simulink model "Third"  (R2021b)
settings: Solver=VariableStepAuto  StartTime=0.0  StopTime=150  RelTol=1e-3
values from neighbouring files (symbols this model uses):
  alpha0 = trim_state_lo(8)    [Glideslope.m]
  coeff_x = x0/sqrt(x0^2+y0^2)    [Glideslope.m]
  coeff_y = y0/sqrt(x0^2+y0^2)    [Glideslope.m]
  h_flare = 19.1817    [Glideslope.m]
  max_dev_elevator = 25 - trim_control_lo(1)    [Glideslope.m]
  max_dev_thrust = 19000 - trim_thrust_lo    [Glideslope.m]
  min_dev_elevator = -25 - trim_control_lo(1)    [Glideslope.m]
  min_dev_thrust = 1000 - trim_thrust_lo    [Glideslope.m]
  tau = 1.2217    [Glideslope.m]
  theta0 = trim_state_lo(5)    [Glideslope.m]
  x0 = 3000 + 2000/(3*pi/180)    (= 41197.1863421)    [Glideslope.m]
undefined symbols (not defined in the file or in its folder): magnitude
libraries: slpidlib x2, cstblocks x1
settings Model: Creator=misha  LastModifiedBy=ddefu

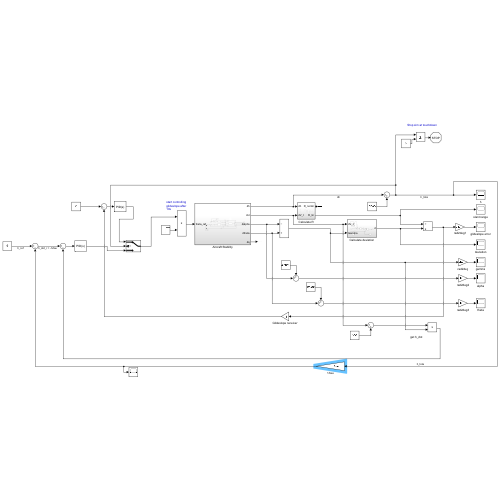
[thumbnail: Simulink's stored preview of the top-level diagram]
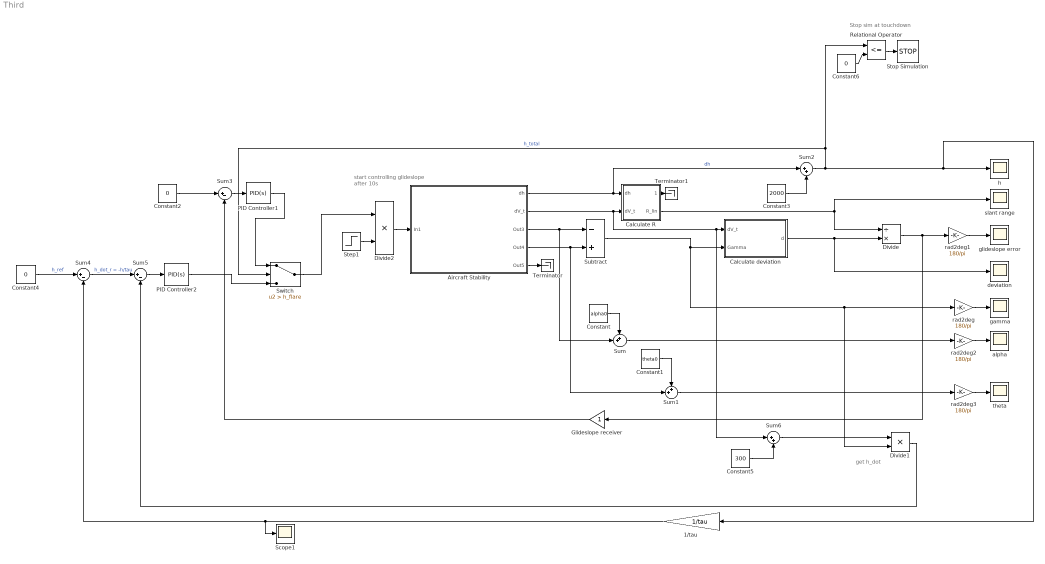
== system Third ==
  note: Stop sim at touchdown
  note: get h_dot
  note: start controlling glideslope after 10s
  1/tau : Gain  Gain=1/tau
  Aircraft Stability : Subsystem
  Calculate R : Subsystem
  Calculate deviation : Subsystem
  Constant : Constant  Value=alpha0
  Constant1 : Constant  Value=theta0
  Constant2 : Constant  Value=0
  Constant3 : Constant  Value=2000
  Constant4 : Constant  Value=0
  Constant5 : Constant  Value=300
  Constant6 : Constant  Value=0
  Divide : Product  Inputs=/*
  Divide1 : Product  Inputs=**
  Divide2 : Product  Inputs=**
  Glideslope receiver : Gain
  PID Controller1 : slpidlib/PID Controller  Controller=PID  Form=Parallel  TimeDomain=Continuous-time  UseExternalTs=off  SampleTime=-1  IntegratorMethod=Forward Euler  FilterMethod=Forward Euler  ControllerParametersSource=internal  P=2000  I=200  D=0  UseFilter=on  N=100  TunerSelectOption=Transfer Function Based (PID Tuner App)  InitialConditionSource=internal  InitialConditionForIntegrator=0  InitialConditionForFilter=0  DifferentiatorICPrevScaledInput=0  ExternalReset=none  TrackingMode=off  Kt=1  LimitOutput=off  SatLimitsSource=internal  UpperSaturationLimit=inf  LowerSaturationLimit=-inf  LinearizeAsGain=on  AntiWindupMode=none  Kb=1  POutMin=[]  POutMax=[]  IOutMin=[]  IOutMax=[]  DOutMin=[]  DOutMax=[]  NOutMin=[]  NOutMax=[]  SumOutMin=[]  SumOutMax=[]  SaturationOutMin=[]  SaturationOutMax=[]  PParamMin=[]  PParamMax=[]  IParamMin=[]  IParamMax=[]  DParamMin=[]  DParamMax=[]  NParamMin=[]  NParamMax=[]  KbParamMin=[]  KbParamMax=[]  KtParamMin=[]  KtParamMax=[]  KbOutMin=[]  KbOutMax=[]  KtOutMin=[]  KtOutMax=[]  IntegratorOutMin=[]  IntegratorOutMax=[]  FilterOutMin=[]  FilterOutMax=[]  SumI1OutMin=[]  SumI1OutMax=[]  SumI2OutMin=[]  SumI2OutMax=[]  SumI3OutMin=[]  SumI3OutMax=[]  SumI4OutMin=[]  SumI4OutMax=[]  SumDOutMin=[]  SumDOutMax=[]  DifferentiatorOutMin=[]  DifferentiatorOutMax=[]  FilterDiffOutCoefMin=[]  FilterDiffOutCoefMax=[]  ReciprocalOutMin=[]  ReciprocalOutMax=[]  SumDenOutMin=[]  SumDenOutMax=[]  SumNumOutMin=[]  SumNumOutMax=[]  DivideOutMin=[]  DivideOutMax=[]  UdiffTsProdOutMin=[]  UdiffTsProdOutMax=[]  NTsProdOutMin=[]  NTsProdOutMax=[]  UintegralTsProdOutMin=[]  UintegralTsProdOutMax=[]  UngainTsProdOutMin=[]  UngainTsProdOutMax=[]  IntegratorContinuousStateAttributes=''  IntegratorStateMustResolveToSignalObject=off  IntegratorRTWStateStorageClass=Auto  FilterContinuousStateAttributes=''  FilterStateMustResolveToSignalObject=off  FilterRTWStateStorageClass=Auto  ParallelPVariant=InternalParameters  IdealPVariant=Disabled  IVariant=InternalParameters  DVariant=InternalParameters  IntegratorVariant=Continuous  SatVariant=Disabled  AWVariant=Passthrough  PCopyVariant=Disabled  TRVariant=Disabled  FdbkBlocksVariant=Forward  IdealPFdbkVariant=Disabled  SatFdbkVariant=Disabled  DerivativeFilterVariant=ContFilter  NVariant=InternalParameters  NCopyVariant=Disabled  FilterICVariant=InternalICsFilter  IntegratorICVariant=InternalICs  ExternalResetVariant=Disabled  TRSumVariant=Passthrough  SumFdbkVariant=Disabled  SumVariant=Sum_PID  TsampFilterVariant=InternalTs  TsampNgainVariant=Passthrough  TsampIntegralVariant=Passthrough  ExternalSaturationOutDataTypeStr=Inherit: Same as second input
  PID Controller2 : slpidlib/PID Controller  Controller=PID  Form=Parallel  TimeDomain=Continuous-time  UseExternalTs=off  SampleTime=-1  IntegratorMethod=Forward Euler  FilterMethod=Forward Euler  ControllerParametersSource=internal  P=2000  I=200  D=0  UseFilter=on  N=100  TunerSelectOption=Transfer Function Based (PID Tuner App)  InitialConditionSource=internal  InitialConditionForIntegrator=0  InitialConditionForFilter=0  DifferentiatorICPrevScaledInput=0  ExternalReset=none  TrackingMode=off  Kt=1  LimitOutput=off  SatLimitsSource=internal  UpperSaturationLimit=inf  LowerSaturationLimit=-inf  LinearizeAsGain=on  AntiWindupMode=none  Kb=1  POutMin=[]  POutMax=[]  IOutMin=[]  IOutMax=[]  DOutMin=[]  DOutMax=[]  NOutMin=[]  NOutMax=[]  SumOutMin=[]  SumOutMax=[]  SaturationOutMin=[]  SaturationOutMax=[]  PParamMin=[]  PParamMax=[]  IParamMin=[]  IParamMax=[]  DParamMin=[]  DParamMax=[]  NParamMin=[]  NParamMax=[]  KbParamMin=[]  KbParamMax=[]  KtParamMin=[]  KtParamMax=[]  KbOutMin=[]  KbOutMax=[]  KtOutMin=[]  KtOutMax=[]  IntegratorOutMin=[]  IntegratorOutMax=[]  FilterOutMin=[]  FilterOutMax=[]  SumI1OutMin=[]  SumI1OutMax=[]  SumI2OutMin=[]  SumI2OutMax=[]  SumI3OutMin=[]  SumI3OutMax=[]  SumI4OutMin=[]  SumI4OutMax=[]  SumDOutMin=[]  SumDOutMax=[]  DifferentiatorOutMin=[]  DifferentiatorOutMax=[]  FilterDiffOutCoefMin=[]  FilterDiffOutCoefMax=[]  ReciprocalOutMin=[]  ReciprocalOutMax=[]  SumDenOutMin=[]  SumDenOutMax=[]  SumNumOutMin=[]  SumNumOutMax=[]  DivideOutMin=[]  DivideOutMax=[]  UdiffTsProdOutMin=[]  UdiffTsProdOutMax=[]  NTsProdOutMin=[]  NTsProdOutMax=[]  UintegralTsProdOutMin=[]  UintegralTsProdOutMax=[]  UngainTsProdOutMin=[]  UngainTsProdOutMax=[]  IntegratorContinuousStateAttributes=''  IntegratorStateMustResolveToSignalObject=off  IntegratorRTWStateStorageClass=Auto  FilterContinuousStateAttributes=''  FilterStateMustResolveToSignalObject=off  FilterRTWStateStorageClass=Auto  ParallelPVariant=InternalParameters  IdealPVariant=Disabled  IVariant=InternalParameters  DVariant=InternalParameters  IntegratorVariant=Continuous  SatVariant=Disabled  AWVariant=Passthrough  PCopyVariant=Disabled  TRVariant=Disabled  FdbkBlocksVariant=Forward  IdealPFdbkVariant=Disabled  SatFdbkVariant=Disabled  DerivativeFilterVariant=ContFilter  NVariant=InternalParameters  NCopyVariant=Disabled  FilterICVariant=InternalICsFilter  IntegratorICVariant=InternalICs  ExternalResetVariant=Disabled  TRSumVariant=Passthrough  SumFdbkVariant=Disabled  SumVariant=Sum_PID  TsampFilterVariant=InternalTs  TsampNgainVariant=Passthrough  TsampIntegralVariant=Passthrough  ExternalSaturationOutDataTypeStr=Inherit: Same as second input
  Relational Operator : RelationalOperator  Operator=<=  OutDataTypeStr=boolean  RndMeth=Simplest
  Scope1 : Scope
  Step1 : Step  Time=10  SampleTime=0
  Stop Simulation : Stop
  Subtract : Sum  Inputs=-+
  Sum : Sum  Inputs=++|
  Sum1 : Sum  Inputs=++|
  Sum2 : Sum  Inputs=|++
  Sum3 : Sum  Inputs=|+-
  Sum4 : Sum  Inputs=|+-
  Sum5 : Sum  Inputs=|+-
  Sum6 : Sum  Inputs=|++
  Switch : Switch  Criteria=u2 > Threshold  Threshold=h_flare
  Terminator : Terminator
  Terminator1 : Terminator
  alpha : Scope
  deviation : Scope
  gamma : Scope
  glideslope error : Scope
  h : Scope
  rad2deg{,1..3} (4 alike) : Gain  Gain=180/pi
  slant range : Scope
  theta : Scope
  wires:
  Aircraft Stability/1(dh) -> Sum2/1, Calculate R/1(dh)  "dh"
  Aircraft Stability/2(dV_t) -> Sum6/1, Calculate deviation/1(dV_t), Calculate R/2(dV_t)
  Aircraft Stability/4(Out4) -> Sum1/2, Subtract/2
  Aircraft Stability/5(Out5) -> Terminator/1
  Divide/1 -> Glideslope receiver/1, rad2deg1/1
  Glideslope receiver/1 -> Sum3/2
  Constant2/1 -> Sum3/1
  Subtract/1 -> Calculate deviation/2(Gamma), rad2deg/1, Divide1/2
  Sum3/1 -> PID Controller1/1
  Aircraft Stability/3(Out3) -> Subtract/1, Sum/2
  PID Controller1/1 -> Switch/1
  Step1/1 -> Divide2/2
  Divide2/1 -> Aircraft Stability/1(In1)
  rad2deg/1 -> gamma/1
  rad2deg1/1 -> glideslope error/1
  Calculate deviation/1(d) -> Divide/2, deviation/1
  Calculate R/1(R_nonlin) -> Terminator1/1
  Calculate R/2(R_lin) -> Divide/1, slant range/1
  Constant/1 -> Sum/1
  Constant1/1 -> Sum1/1
  rad2deg2/1 -> alpha/1
  rad2deg3/1 -> theta/1
  Sum/1 -> rad2deg2/1
  Sum1/1 -> rad2deg3/1
  Constant3/1 -> Sum2/2
  Sum2/1 -> Relational Operator/1, Switch/2, 1/tau/1, h/1  "h_total"
  Constant4/1 -> Sum4/1  "h_ref"
  1/tau/1 -> Scope1/1, Sum4/2
  Sum4/1 -> Sum5/1  "h_dot_r = -h/tau"
  Constant5/1 -> Sum6/2
  Sum6/1 -> Divide1/1
  Divide1/1 -> Sum5/2
  Sum5/1 -> PID Controller2/1
  Relational Operator/1 -> Stop Simulation/1
  Constant6/1 -> Relational Operator/2
  Switch/1 -> Divide2/1
  PID Controller2/1 -> Switch/3

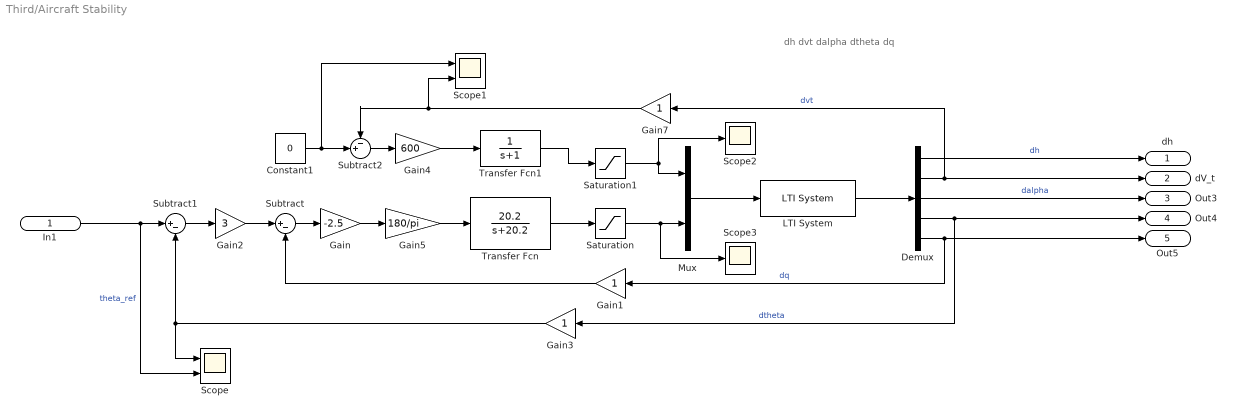
== system Third/Aircraft Stability ==
  note: dh
      | dvt
      | dalpha
      | dtheta
      | dq
  In1 : Inport
  Constant1 : Constant  Value=0
  Demux : Demux  Outputs=5
  Gain : Gain  Gain=-2.5
  Gain1 : Gain
  Gain2 : Gain  Gain=3
  Gain3 : Gain
  Gain4 : Gain  Gain=600
  Gain5 : Gain  Gain=180/pi
  Gain7 : Gain
  LTI System : cstblocks/LTI System  sys=sys_reduced  IC=[]
  Mux : Mux  Inputs=2
  Saturation : Saturate  UpperLimit=max_dev_elevator  LowerLimit=min_dev_elevator
  Saturation1 : Saturate  UpperLimit=max_dev_thrust  LowerLimit=min_dev_thrust
  Scope : Scope  NumInputPorts=2
  Scope1 : Scope  NumInputPorts=2
  Scope2 : Scope
  Scope3 : Scope
  Subtract : Sum  Inputs=|+-
  Subtract1 : Sum  Inputs=|+-
  Subtract2 : Sum  Inputs=-+|
  Transfer Fcn : TransferFcn  Numerator=[20.2]  Denominator=[1 20.2]
  Transfer Fcn1 : TransferFcn  Denominator=[1 1]
  dh : Outport
  dV_t : Outport  Port=2
  Out3 : Outport  Port=3
  Out4 : Outport  Port=4
  Out5 : Outport  Port=5
  wires:
  Gain5/1 -> Transfer Fcn/1
  In1/1 -> Subtract1/1, Scope/2  "theta_ref"
  Demux/4 -> Out4/1, Gain3/1  "dtheta"
  Gain2/1 -> Subtract/1
  Gain/1 -> Gain5/1
  Mux/1 -> LTI System/1
  Gain1/1 -> Subtract/2
  Gain3/1 -> Subtract1/2, Scope/1
  Saturation/1 -> Mux/2, Scope3/1
  Transfer Fcn1/1 -> Saturation1/1
  LTI System/1 -> Demux/1
  Saturation1/1 -> Scope2/1, Mux/1
  Demux/3 -> Out3/1  "dalpha"
  Demux/2 -> dV_t/1, Gain7/1  "dvt"
  Demux/5 -> Gain1/1, Out5/1  "dq"
  Subtract/1 -> Gain/1
  Constant1/1 -> Scope1/1, Subtract2/2
  Gain7/1 -> Scope1/2, Subtract2/1
  Demux/1 -> dh/1  "dh"
  Subtract1/1 -> Gain2/1
  Transfer Fcn/1 -> Saturation/1
  Subtract2/1 -> Gain4/1
  Gain4/1 -> Transfer Fcn1/1

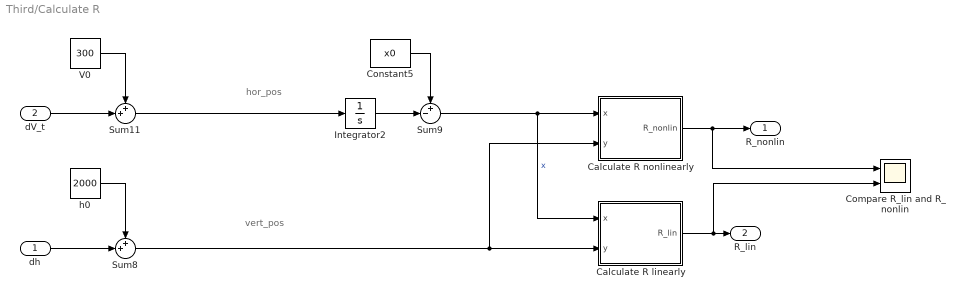
== system Third/Calculate R ==
  note: vert_pos
  note: hor_pos
  dh : Inport
  dV_t : Inport  Port=2
  Calculate R linearly : Subsystem
  Calculate R nonlinearly : Subsystem
  Compare R_lin and R_nonlin : Scope  NumInputPorts=2
  Constant5 : Constant  Value=x0
  Integrator2 : Integrator
  Sum11 : Sum  Inputs=++|
  Sum8 : Sum  Inputs=++|
  Sum9 : Sum  Inputs=+-|
  V0 : Constant  Value=300
  h0 : Constant  Value=2000
  R_nonlin : Outport
  R_lin : Outport  Port=2
  wires:
  Sum8/1 -> Calculate R linearly/2(y), Calculate R nonlinearly/2(y)
  Sum9/1 -> Calculate R linearly/1(x), Calculate R nonlinearly/1(x)  "x"
  dh/1 -> Sum8/2
  dV_t/1 -> Sum11/2
  h0/1 -> Sum8/1
  Integrator2/1 -> Sum9/2
  Sum11/1 -> Integrator2/1
  Constant5/1 -> Sum9/1
  V0/1 -> Sum11/1
  Calculate R linearly/1(R_lin) -> Compare R_lin and R_nonlin/2, R_lin/1
  Calculate R nonlinearly/1(R_nonlin) -> Compare R_lin and R_nonlin/1, R_nonlin/1

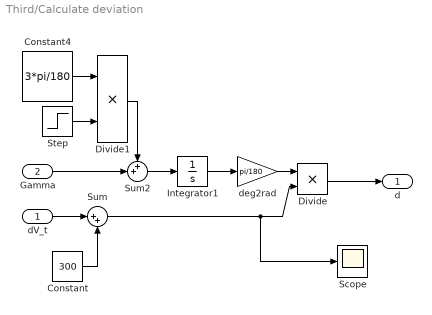
== system Third/Calculate deviation ==
  dV_t : Inport
  Gamma : Inport  Port=2
  Constant : Constant  Value=300
  Constant4 : Constant  Value=3*pi/180
  Divide : Product  Inputs=**
  Divide1 : Product  Inputs=**
  Integrator1 : Integrator
  Scope : Scope
  Step : Step  Time=10  SampleTime=0
  Sum : Sum  Inputs=|++
  Sum2 : Sum  Inputs=++|
  deg2rad : Gain  Gain=pi/180
  d : Outport
  wires:
  Constant4/1 -> Divide1/1
  Sum2/1 -> Integrator1/1
  Gamma/1 -> Sum2/2
  Integrator1/1 -> deg2rad/1
  Step/1 -> Divide1/2
  Divide1/1 -> Sum2/1
  dV_t/1 -> Sum/1
  Constant/1 -> Sum/2
  Divide/1 -> d/1
  deg2rad/1 -> Divide/1
  Sum/1 -> Scope/1, Divide/2

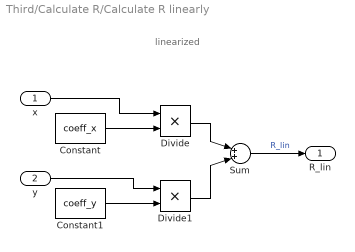
== system Third/Calculate R/Calculate R linearly ==
  note: linearized
  x : Inport
  y : Inport  Port=2
  Constant : Constant  Value=coeff_x
  Constant1 : Constant  Value=coeff_y
  Divide : Product  Inputs=**
  Divide1 : Product  Inputs=**
  Sum : Sum  Inputs=|++|
  R_lin : Outport
  wires:
  y/1 -> Divide1/1
  Constant1/1 -> Divide1/2
  Divide/1 -> Sum/1
  Divide1/1 -> Sum/2
  Constant/1 -> Divide/2
  Sum/1 -> R_lin/1  "R_lin"
  x/1 -> Divide/1

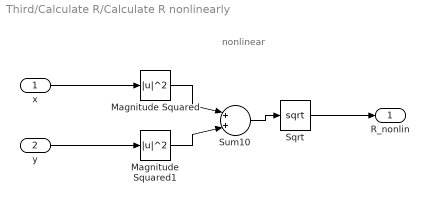
== system Third/Calculate R/Calculate R nonlinearly ==
  note: nonlinear
  x : Inport
  y : Inport  Port=2
  Magnitude Squared : Math  Operator=magnitude^2  SaturateOnIntegerOverflow=on
  Magnitude Squared1 : Math  Operator=magnitude^2  SaturateOnIntegerOverflow=on
  Sqrt : Sqrt  SaturateOnIntegerOverflow=on
  Sum10 : Sum  Inputs=|++|
  R_nonlin : Outport
  wires:
  Magnitude Squared/1 -> Sum10/1
  Magnitude Squared1/1 -> Sum10/2
  Sum10/1 -> Sqrt/1
  Sqrt/1 -> R_nonlin/1
  x/1 -> Magnitude Squared/1
  y/1 -> Magnitude Squared1/1
